simulink model "DT_DSM_CRFB_LOWPASS_2nd_2048"  (R2025b)
settings: Solver=VariableStepAuto  StartTime=0.0  StopTime=1  RelTol=1e-3
libraries: simulink_extras x1
settings Model: Creator=Team_33  LastModifiedBy=k2vas

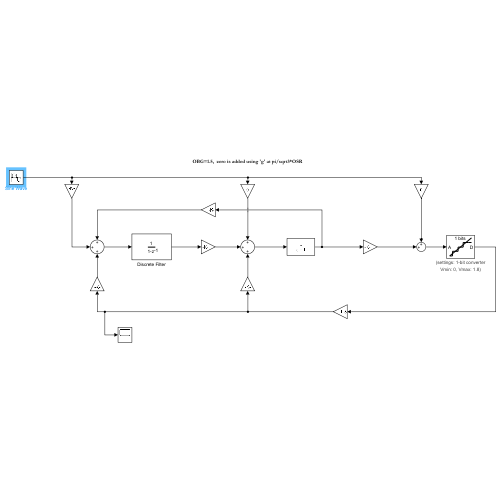
[thumbnail: Simulink's stored preview of the top-level diagram]
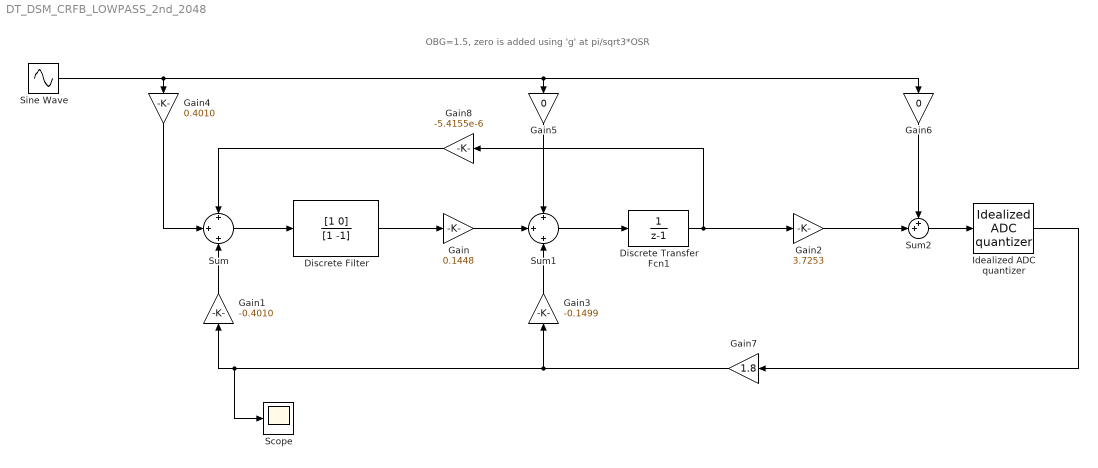
== system DT_DSM_CRFB_LOWPASS_2nd_2048 ==
  note: OBG=1.5, zero is added using 'g' at pi/sqrt3*OSR
  Discrete Transfer Fcn1 : DiscreteTransferFcn  Denominator=[1 -1]
  Discrete Filter : DiscreteFilter  Numerator=[1 0]  Denominator=[1 -1]  InputProcessing=Columns as channels (frame based)  FilterStructure=Direct form II transposed  a0EqualsOne=on
  Gain : Gain  Gain=0.1448
  Gain1 : Gain  Gain=-0.4010
  Gain2 : Gain  Gain=3.7253
  Gain3 : Gain  Gain=-0.1499
  Gain4 : Gain  Gain=0.4010
  Gain5 : Gain  Gain=0
  Gain6 : Gain  Gain=0
  Gain7 : Gain  Gain=1.8
  Gain8 : Gain  Gain=-5.4155e-6
  Idealized ADC quantizer : simulink_extras/Additional Discrete/Idealized ADC quantizer  NumberOfConverterBits=1  Vmin=0  Vmax=1.8  OutputDataType=int32  OutputNegativeValues=off
  Scope : Scope
      settings: ActiveDisplayYMinimum=-0.17789  ActiveDisplayYMaximum=1.87446  DataLoggingVariableName=output_data  DataLoggingSaveFormat=Array
  Sine Wave : Sin  Amplitude=0.6  Bias=0.9  Frequency=((2000*2048)*127*2*pi)/(32768*32)  SampleTime=1/(2000*2048)
  Sum : Sum  Inputs=+|+|+
  Sum1 : Sum  Inputs=+|+|+
  Sum2 : Sum  Inputs=++|
  wires:
  Sum1/1 -> Discrete Transfer Fcn1/1
  Discrete Transfer Fcn1/1 -> Gain8/1, Gain2/1
  Gain4/1 -> Sum/2
  Gain1/1 -> Sum/3
  Gain/1 -> Sum1/2
  Gain3/1 -> Sum1/3
  Gain2/1 -> Sum2/2
  Gain5/1 -> Sum1/1
  Gain6/1 -> Sum2/1
  Sum2/1 -> Idealized ADC quantizer/1
  Sine Wave/1 -> Gain6/1, Gain5/1, Gain4/1
  Idealized ADC quantizer/1 -> Gain7/1
  Gain8/1 -> Sum/1
  Discrete Filter/1 -> Gain/1
  Gain7/1 -> Scope/1, Gain1/1, Gain3/1
  Sum/1 -> Discrete Filter/1
